simulink model "dspenvdet"  (Simulink 8.3)
settings: Solver=FixedStepDiscrete  StartTime=0.0  StopTime=4.99  RelTol=1e-3
PreLoadFcn:
  | load('speech_dft')
values from neighbouring files (symbols this model uses):
  fs = AudioInput.SampleRate    [AudioArrayDOAEstimationExample.m]    (also in HelperDesa2Sysobj.m = 500; HelperDesa2SysobjTestBLNG.m = 500)
undefined symbols (not defined in the file or in its folder): dfilt, Newton, Raphson
libraries: dsparch4 x3, dspsrcs4 x2, dspmlti4 x2, dspsigops x1, dspmisc x1
CloseFcn:
  | clear fs;clear y; clear tout
settings Model: Creator=The MathWorks Inc.  ExtModeAutoUpdateStatusClock=off
settings OptimizationCC: ExpressionDepthLimit=2147483647  InitFltsAndDblsToZero=on
settings DebuggingCC: SaveWithParameterizedLinksMsg=none  SignalResolutionControl=TryResolveAllWithWarning  SolverPrmCheckMsg=none  MultiTaskDSMMsg=warning  MultiTaskCondExecSysMsg=none  SigSpecEnsureSampleTimeMsg=none  FcnCallInpInsideContextMsg=UseLocalSettings  StrictBusMsg=Warning
settings RTWCC: IncludeERTFirstTime=on
settings GRTTargetCC: TargetFcnLib=ansi_tfl_tmw.mat

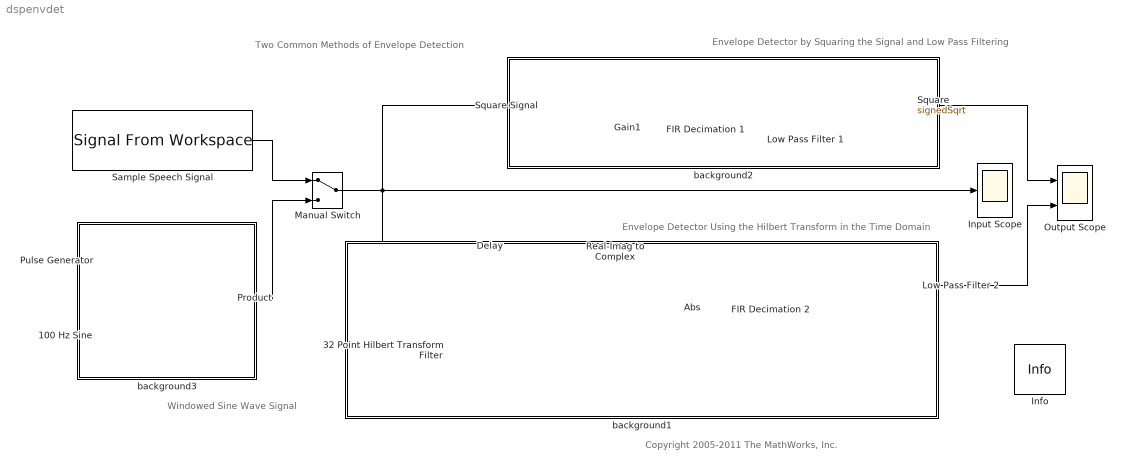
== system dspenvdet ==
  note: Envelope Detector Using the Hilbert Transform in the Time Domain
  note: Two Common Methods of Envelope Detection
  note: Envelope Detector by Squaring the Signal and Low Pass Filtering
  note: Windowed Sine Wave Signal
  note: Copyright 2005-2011 The MathWorks, Inc.
  100 Hz Sine : dspsrcs4/Sine Wave  Amplitude=1  Frequency=100  Phase=0  SampleMode=Discrete  OutComplex=Real  CompMethod=Trigonometric fcn  TableSize=Speed  SampleTime=1/22050  SamplesPerFrame=1  ResetState=Restart at time zero  dataType=double  wordLen=16  udDataType=sfix(16)  fracBitsMode=Best precision  numFracBits=15  OutDataTypeStr=double  LastOutDataTypeStr=double
  32 Point Hilbert Transform Filter : dsparch4/Digital Filter  TypePopup=FIR (all zeros)  IIRFiltStruct=Direct form II transposed  AllPoleFiltStruct=Direct form  FIRFiltStruct=Direct form  CoeffSource=Specify via dialog  NumCoeffs=firpm(32, [0.1 0.9], [1 1], 'hilbert')  DenCoeffs=[1 0.1]  BiQuadCoeffs=[1 0.3 0.4 1 0.1 0.2]  LatticeCoeffs=[0.2 0.4]  denIgnore=on  FiltPerSampPopup=One filter per frame  IC=0  ICnum=0  ICden=0  roundingMode=Floor  overflowMode=off  ScaleValues=1  scaleValueFracLength=14  stageInFracLength=15  stageOutFracLength=15  FilterSource=Specify via dialog  dfiltObjectName=dfilt.dffir([1 2 1])
  Abs : Abs
  Delay : dspsigops/Delay  dly_unit=Samples  delay=16  ic_detail=off  dif_ic_for_ch=off  dif_ic_for_dly=off  ic=0  reset_popup=None
  FIR Decimation 1 : dspmlti4/FIR Decimation  h=[1 1]  D=15  filtStruct=Direct form  framing=Maintain input frame size  inputOffset=0  outputBufInitCond=0  firstCoeffDataTypeStr=Inherit: Same word length as input  firstCoeffLastDataTypeStr=Inherit: Same word length as input  firstCoeffMin=[]  firstCoeffMax=[]  outputMin=[]  outputMax=[]  roundingMode=Floor  overflowMode=off  FilterSource=Specify via dialog  FilterObject=Hm_firdecim
  FIR Decimation 2 : dspmlti4/FIR Decimation  h=[1 1]  D=15  filtStruct=Direct form  framing=Maintain input frame size  inputOffset=0  outputBufInitCond=0  firstCoeffDataTypeStr=Inherit: Same word length as input  firstCoeffLastDataTypeStr=Inherit: Same word length as input  firstCoeffMin=[]  firstCoeffMax=[]  outputMin=[]  outputMax=[]  roundingMode=Floor  overflowMode=off  FilterSource=Specify via dialog  FilterObject=Hm_firdecim
  Gain1 : Gain  Gain=2
  Info : dspmisc/Info  SystemSampleTime=-1
  Input Scope : Scope
      settings: TimeRange=1  YMin=-1  YMax=1  MaxDataPoints=22050
  Low Pass Filter 1 : dsparch4/Digital Filter  TypePopup=FIR (all zeros)  IIRFiltStruct=Direct form II transposed  AllPoleFiltStruct=Direct form  FIRFiltStruct=Direct form  CoeffSource=Specify via dialog  NumCoeffs=firpm(20, [0 0.03 0.1 1], [1 1 0 0])  DenCoeffs=1  BiQuadCoeffs=[1 0.3 0.4 1 0.1 0.2]  LatticeCoeffs=[0.2 0.4]  denIgnore=on  FiltPerSampPopup=One filter per frame  IC=0  ICnum=0  ICden=0  roundingMode=Floor  overflowMode=off  ScaleValues=1  scaleValueFracLength=14  stageInFracLength=15  stageOutFracLength=15  FilterSource=Specify via dialog  dfiltObjectName=dfilt.dffir([1 2 1])
  Low Pass Filter 2 : dsparch4/Digital Filter  TypePopup=FIR (all zeros)  IIRFiltStruct=Direct form II transposed  AllPoleFiltStruct=Direct form  FIRFiltStruct=Direct form  CoeffSource=Specify via dialog  NumCoeffs=firpm(20, [0 0.03 0.1 1], [1 1 0 0])  DenCoeffs=1  BiQuadCoeffs=[1 0.3 0.4 1 0.1 0.2]  LatticeCoeffs=[0.2 0.4]  denIgnore=on  FiltPerSampPopup=One filter per frame  IC=0  ICnum=0  ICden=0  roundingMode=Floor  overflowMode=off  ScaleValues=1  scaleValueFracLength=14  stageInFracLength=15  stageOutFracLength=15  FilterSource=Specify via dialog  dfiltObjectName=dfilt.dffir([1 2 1])
  Manual Switch : ManualSwitch
  Output Scope : Scope  NumInputPorts=2
      settings: TimeRange=1  YMin=-1~-1  YMax=1~1  MaxDataPoints=22050
  Product : Product  RndMeth=Zero
  Pulse Generator : DiscretePulseGenerator  Amplitude=0.5  Period=7000  PulseWidth=4000  SampleTime=1/22050
  Real-Imag to Complex : RealImagToComplex
  Sample Speech Signal : dspsrcs4/Signal From Workspace  X=y  Ts=1/fs  nsamps=1  OutputAfterFinalValue=Setting to zero  ignoreOrWarnInputAndFrameLengths=off
  "Square " : Sqrt  Operator=signedSqrt  AlgorithmType=Newton-Raphson  SaturateOnIntegerOverflow=on
  Square Signal : Math  Operator=square  SaturateOnIntegerOverflow=on
  background1 : Subsystem
      mask Display: disp('');
  background2 : Subsystem
      mask Display: disp('')
  background3 : Subsystem
      mask Display: disp('')
  wires:
  32 Point Hilbert Transform Filter/1 -> Real-Imag to Complex/2
  Abs/1 -> FIR Decimation 2/1
  Square Signal/1 -> Gain1/1
  Gain1/1 -> FIR Decimation 1/1
  Low Pass Filter 1/1 -> "Square "/1
  FIR Decimation 1/1 -> Low Pass Filter 1/1
  FIR Decimation 2/1 -> Low Pass Filter 2/1
  Manual Switch/1 -> Square Signal/1, 32 Point Hilbert Transform Filter/1, Delay/1, Input Scope/1
  Sample Speech Signal/1 -> Manual Switch/1
  Pulse Generator/1 -> Product/1
  100 Hz Sine/1 -> Product/2
  Product/1 -> Manual Switch/2
  "Square "/1 -> Output Scope/1
  Low Pass Filter 2/1 -> Output Scope/2
  Delay/1 -> Real-Imag to Complex/1
  Real-Imag to Complex/1 -> Abs/1

== system dspenvdet/background1 ==

== system dspenvdet/background2 ==

== system dspenvdet/background3 ==
